simulink library "csc_gdn_guidance_mtv_lib"  (R2014b)
settings: Solver=ode45  StartTime=0.0  StopTime=10.0  RelTol=1e-3
undefined symbols (not defined in the file or in its folder): csc_gdn_dt
libraries: util_info_lib x1, csc_cgs_coast_guidance_system_mtv_lib x1, csc_gal_gdn_approach_landing_mtv_lib x1, csc_gib_gdn_inertial_burn_mtv_lib x1, csu_gml_guidance_mode_logic_lib x1
settings Model: Creator=Nilesh  LastModifiedBy=tgorton

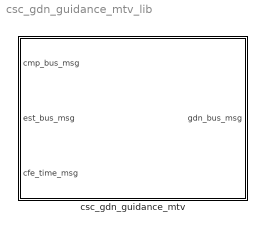
== system csc_gdn_guidance_mtv_lib ==
  csc_gdn_guidance_mtv : Subsystem  Tag=OFSW; MDL_TICK=EST_BUS_MSG  TreatAsAtomicUnit=on  SystemSampleTime=csc_gdn_dt

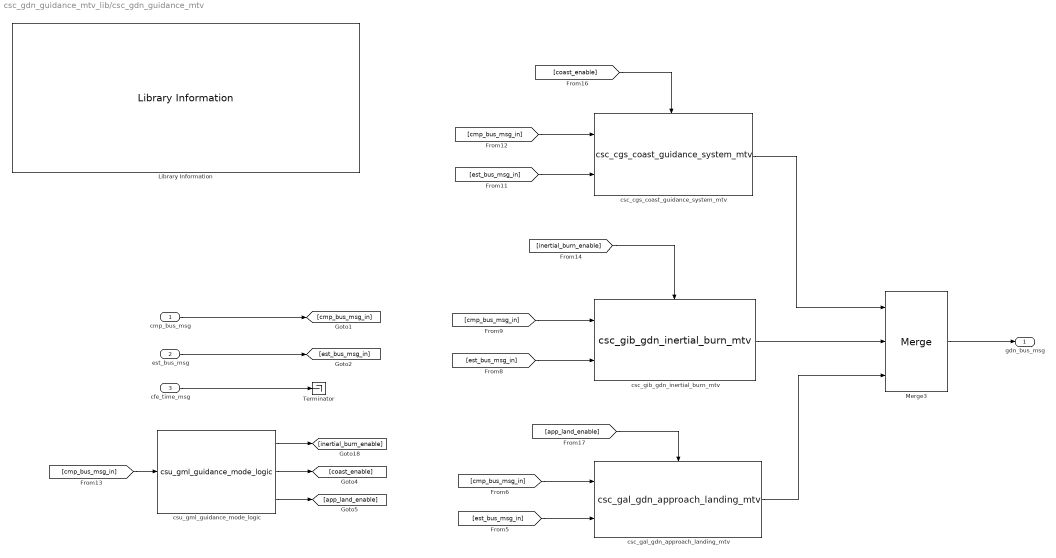
== system csc_gdn_guidance_mtv_lib/csc_gdn_guidance_mtv ==
  cmp_bus_msg : Inport
  est_bus_msg : Inport  Port=2
  cfe_time_msg : Inport  Port=3  OutDataTypeStr=Bus: cfe_time_msg
  Library Information : util_info_lib/Library Information  owner='jkaidy'
  Merge3 : Merge  Inputs=3  InitialOutput=0
  Terminator : Terminator
  csc_cgs_coast_guidance_system_mtv : csc_cgs_coast_guidance_system_mtv_lib/csc_cgs_coast_guidance_system_mtv
  csc_gal_gdn_approach_landing_mtv : csc_gal_gdn_approach_landing_mtv_lib/csc_gal_gdn_approach_landing_mtv
  csc_gib_gdn_inertial_burn_mtv : csc_gib_gdn_inertial_burn_mtv_lib/csc_gib_gdn_inertial_burn_mtv
  csu_gml_guidance_mode_logic : csu_gml_guidance_mode_logic_lib/csu_gml_guidance_mode_logic
  gdn_bus_msg : Outport  OutDataTypeStr=Bus: gdn_bus_msg
  wires:
  cfe_time_msg/1 -> Terminator/1
  csc_gal_gdn_approach_landing_mtv/1 -> Merge3/3
  csu_gml_guidance_mode_logic/1 -> [inertial_burn_enable]
  cmp_bus_msg/1 -> [cmp_bus_msg_in]
  est_bus_msg/1 -> [est_bus_msg_in]
  [est_bus_msg_in] -> csc_gal_gdn_approach_landing_mtv/2
  [cmp_bus_msg_in] -> csc_gal_gdn_approach_landing_mtv/1
  [cmp_bus_msg_in] -> csc_gib_gdn_inertial_burn_mtv/1
  [est_bus_msg_in] -> csc_gib_gdn_inertial_burn_mtv/2
  [cmp_bus_msg_in] -> csc_cgs_coast_guidance_system_mtv/1
  [est_bus_msg_in] -> csc_cgs_coast_guidance_system_mtv/2
  csu_gml_guidance_mode_logic/2 -> [coast_enable]
  csu_gml_guidance_mode_logic/3 -> [app_land_enable]
  [cmp_bus_msg_in] -> csu_gml_guidance_mode_logic/1
  [app_land_enable] -> csc_gal_gdn_approach_landing_mtv/Enable
  [inertial_burn_enable] -> csc_gib_gdn_inertial_burn_mtv/Enable
  [coast_enable] -> csc_cgs_coast_guidance_system_mtv/Enable
  csc_gib_gdn_inertial_burn_mtv/1 -> Merge3/2
  csc_cgs_coast_guidance_system_mtv/1 -> Merge3/1
  Merge3/1 -> gdn_bus_msg/1
